simulink model "Model_HeliCE150_PID_FFCwithNN"  (R2020b)
settings: Solver=FixedStepAuto  StartTime=0.0  StopTime=200  FixedStep=1e-2  RelTol=1e-3
values from neighbouring files (symbols this model uses):
  a_1 = 0.105    [Main_HeliCE150_PID_FFCwithNN.m]    (also in Param_HeliCE150_PID_FFCwithNN.m)
  a_2 = 0.033    [Main_HeliCE150_PID_FFCwithNN.m]    (also in Param_HeliCE150_PID_FFCwithNN.m)
  b_1 = 0.00936    [Main_HeliCE150_PID_FFCwithNN.m]    (also in Param_HeliCE150_PID_FFCwithNN.m)
  b_2 = 0.0294    [Main_HeliCE150_PID_FFCwithNN.m]    (also in Param_HeliCE150_PID_FFCwithNN.m)
  B_phi = 0.00869    [Main_HeliCE150_PID_FFCwithNN.m]    (also in Param_HeliCE150_PID_FFCwithNN.m)
  B_psi = 0.00184    [Main_HeliCE150_PID_FFCwithNN.m]    (also in Param_HeliCE150_PID_FFCwithNN.m)
  desired_phi = 2    [Main_HeliCE150_PID_FFCwithNN.m]
  desired_psi = 2    [Main_HeliCE150_PID_FFCwithNN.m]
  dirIn = 2    [Main_HeliCE150_PID_FFCwithNN.m]
  dirIn_switch = 0    [Main_HeliCE150_PID_FFCwithNN.m]
  FFC_switch = 1    [Main_HeliCE150_PID_FFCwithNN.m]
  FFC_u1_net = 4    [Main_HeliCE150_PID_FFCwithNN.m]
  FFC_u2_net = 3    [Main_HeliCE150_PID_FFCwithNN.m]
  fixPhi = 0    [Main_HeliCE150_PID_FFCwithNN.m]
  I = 0.00437    [Main_HeliCE150_PID_FFCwithNN.m]    (also in Param_HeliCE150_PID_FFCwithNN.m)
  I_phi = 0.00414    [Main_HeliCE150_PID_FFCwithNN.m]    (also in Param_HeliCE150_PID_FFCwithNN.m)
  K_Gyro = 0.015    [Main_HeliCE150_PID_FFCwithNN.m]    (also in Param_HeliCE150_PID_FFCwithNN.m)
  K_r = 0.00162    [Main_HeliCE150_PID_FFCwithNN.m]    (also in Param_HeliCE150_PID_FFCwithNN.m)
  PID_u1_switch = 1    [Main_HeliCE150_PID_FFCwithNN.m]
  PID_u2_switch = 1    [Main_HeliCE150_PID_FFCwithNN.m]
  T_0r = 2.7    [Main_HeliCE150_PID_FFCwithNN.m]    (also in Param_HeliCE150_PID_FFCwithNN.m)
  T_1 = 0.3    [Main_HeliCE150_PID_FFCwithNN.m]    (also in Param_HeliCE150_PID_FFCwithNN.m)
  T_2 = 0.25    [Main_HeliCE150_PID_FFCwithNN.m]    (also in Param_HeliCE150_PID_FFCwithNN.m)
  T_pr = 0.75    [Main_HeliCE150_PID_FFCwithNN.m]    (also in Param_HeliCE150_PID_FFCwithNN.m)
  T_u1 = 0    [Main_HeliCE150_PID_FFCwithNN.m]    (also in Param_HeliCE150_PID_FFCwithNN.m)
  T_u2 = 1    [Main_HeliCE150_PID_FFCwithNN.m]    (also in Param_HeliCE150_PID_FFCwithNN.m)
  Tau_g = 0.0383    [Main_HeliCE150_PID_FFCwithNN.m]    (also in Param_HeliCE150_PID_FFCwithNN.m)
libraries: neural x56, pid_lib x3, simulink x2
(part 4 of 4)

== system Model_HeliCE150_PID_FFCwithNN/Feedback Control with PID + Feedforward Compensation with Neural Networks/FFNet - Single Layer Perceptor [5] In: [psi_d] // Out: [u_1]/Layer 2/LW{2,1} ==
  "ad{2,1}" : Inport  PortDimensions=5
      mask Display: e = 0.06;c1 = [120 230 180]/255;c2 = ([120 230 180]+0)/(256+128);c3 = ([120 230 180]+128)/(256+128);patch([0 1 1 0],[0 0 1 1],c1);patch([0 1 1 1-e 1-e 0+e],[0 0 1 1-e 0+e 0+e],c2);patch([0 0 1 1-e 0+e 0+e],[0 1 1 1-e 1-e 0+e],c3);plot([0 1 1 0 0],[0 0 1 1 0]);
  "IW{2,1}(1,:)'" : Constant  Value=[0.0268853418021881840349607273310539312660694122314453125;0.0179021802413151069621743971538307960145175457000732421875;-0.703921131242669417815704946406185626983642578125;0.281780685765841643064533172946539707481861114501953125;-0.1298379463283738377565867949670064263045787811279296875]
      mask Display: e = 0.06;c1 = [120 150 230]/255;c2 = ([120 150 230]+0)/383;c3 = ([120 150 230]+128)/383;patch([0 1 1 0],[0 0 1 1],c1);patch([0 1 1 1-e 1-e 0+e],[0 0 1 1-e 0+e 0+e],c2);patch([0 0 1 1-e 0+e 0+e],[0 1 1 1-e 1-e 0+e],c3);plot([0 1 1 0 0],[0 0 1 1 0]);disp('weights');
  Mux : Mux  Inputs=1
      mask Display: e = 0.06;c1 = [120 150 230]/255;c2 = ([120 150 230]+0)/383;c3 = ([120 150 230]+128)/383;patch([0 1 1 0],[0 0 1 1],c1);patch([0 1 1 1-e 1-e 0+e],[0 0 1 1-e 0+e 0+e],c2);patch([0 0 1 1-e 0+e 0+e],[0 1 1 1-e 1-e 0+e],c3);plot([0 1 1 0 0],[0 0 1 1 0]);disp('Mux');
  dotprod1 : neural/Weight Functions/dotprod
  "lz{2,1}" : Outport
      mask Display: e = 0.06;c1 = [120 230 180]/255;c2 = ([120 230 180]+0)/(256+128);c3 = ([120 230 180]+128)/(256+128);patch([0 1 1 0],[0 0 1 1],c1);patch([0 1 1 1-e 1-e 0+e],[0 0 1 1-e 0+e 0+e],c2);patch([0 0 1 1-e 0+e 0+e],[0 1 1 1-e 1-e 0+e],c3);plot([0 1 1 0 0],[0 0 1 1 0]);
  wires:
  "IW{2,1}(1,:)'"/1 -> dotprod1/1
  "ad{2,1}"/1 -> dotprod1/2
  dotprod1/1 -> Mux/1
  Mux/1 -> "lz{2,1}"/1

== matlab function Model_HeliCE150_PID_FFCwithNN/Feedback Control with PID + Feedforward Compensation with Neural Networks/Psi <45°,88°> ==
  data: PID input; u1 output; err input; psi_d input; sig output
function [u1, sig] = fcn(PID,err,psi_d)
sig = 0;
u1 = 0;
if err < 1.5 && err > 1 && psi_d < 88
    u1 = PID;
end

if psi_d >=88
    sig = 1;
end
